simulink model "StateRequest"  (R2024a)
settings: Solver=FixedStepDiscrete  StartTime=0.0  StopTime=20  FixedStep=.005  RelTol=1e-3
values from neighbouring files (symbols this model uses):
  PrimaryState : value not decoded    [Dictionary.sldd]
libraries: simulink x4
settings Model: DataDictionary=Dictionary.sldd  Creator=aloehr  LastModifiedBy=aloehr
settings SolverCC: AlgebraicLoopSolver=TrustRegion  PositivePriorityOrder=on
settings OptimizationCC: DefaultParameterBehavior=Inlined  UseDivisionForNetSlopeComputation=on  GainParamInheritBuiltInType=on  UseFloatMulNetSlope=on  DefaultUnderspecifiedDataType=single  InlineInvariantSignals=on  PassReuseOutputArgsAs=Individual arguments  ZeroExternalMemoryAtStartup=off  ZeroInternalMemoryAtStartup=off  NoFixptDivByZeroProtection=on  EfficientFloat2IntCast=on  LifeSpan=1  MaxStackSize=64  OptimizeBlockOrder=speed  DifferentSizesBufferReuse=on  EfficientTunableParamExpr=on
settings DebuggingCC: ParameterTunabilityLossMsg=error  UnconnectedInputMsg=warning  UnconnectedOutputMsg=warning  UnconnectedLineMsg=warning  SFUnexpectedBacktrackingDiag=warning  SFNoUnconditionalDefaultTransitionDiag=warning
settings HardwareCC: ProdBitPerPointer=32  ProdBitPerSizeT=32  ProdBitPerPtrDiffT=32  ProdLargestAtomicInteger=Long  ProdLargestAtomicFloat=Double  ProdWordSize=32  ProdLongLongMode=on  ProdHWDeviceType=ARM Compatible->ARM Cortex-M  TargetBitPerPointer=64  TargetBitPerSizeT=64  TargetBitPerPtrDiffT=64  TargetLongLongMode=on  TargetIntDivRoundTo=Zero  TargetEndianess=LittleEndian  TargetWordSize=64  TargetHWDeviceType=MATLAB Host  ProdEqTarget=off
settings ModelReferenceCC: EnableRefExpFcnMdlSchedulingChecks=on
settings SFSimCC: MATLABDynamicMemAlloc=off
settings RTWCC: Description=Embedded Coder  SystemTargetFile=ert.tlc  GenCodeOnly=on  TemplateMakefile=ert_default_tmf  GenerateReport=on  Toolchain=GNU Tools for ARM Embedded Processors  BuildConfiguration=Debug  IncludeHyperlinkInReport=on  LaunchReport=on  DataTypeReplacement=CDataTypesFixedWidth  GenerateTraceInfo=on  GenerateTraceReport=on  GenerateTraceReportSl=on  GenerateTraceReportSf=on  GenerateTraceReportEml=on  GenerateCodeMetricsReport=on  GPUComputeCapability=3.5
settings CodeAppCC: ForceParamTrailComments=on  IgnoreCustomStorageClasses=off  OperatorAnnotations=on  SimulinkDataObjDesc=on  SFDataObjDesc=on  CustomSymbolStrGlobalVar=rt$N$M  CustomSymbolStrType=$N$M  CustomSymbolStrFcn=$N$M$F  CustomSymbolStrMacro=$N$M  InsertBlockDesc=on  EnableCustomComments=on  ReqsInCode=on
settings ERTTargetCC: TargetLangStandard=C99 (ISO)  CodeReplacementLibrary=GNU C99 extensions  GenerateSampleERTMain=on  IncludeMdlTerminateFcn=off  CombineSignalStateStructs=on  SupportAbsoluteTime=off  CodeInterfacePackaging=Reusable function  SupportComplex=off  SupportNonInlinedSFcns=on  InlinedParameterPlacement=NonHierarchical  ERTCustomFileTemplate=example_file_process.tlc  MaxIdInt64=INT64_MAX  MinIdInt64=INT64_MIN  MaxIdUint64=UINT64_MAX  MaxIdInt32=INT32_MAX  MinIdInt32=INT32_MIN  MaxIdUint32=UINT32_MAX  MaxIdInt16=INT16_MAX  MinIdInt16=INT16_MIN  MaxIdUint16=UINT16_MAX  MaxIdInt8=INT8_MAX  MinIdInt8=INT8_MIN  MaxIdUint8=UINT8_MAX

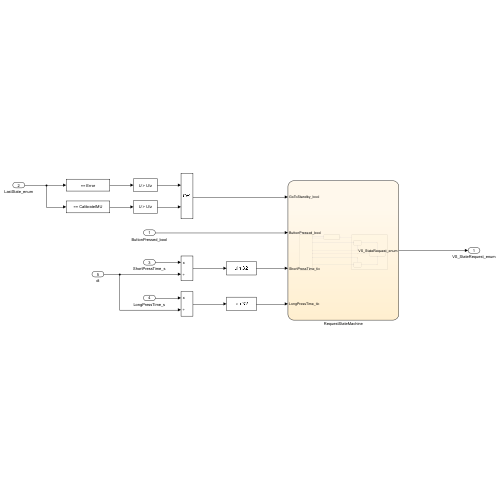
[thumbnail: Simulink's stored preview of the top-level diagram]
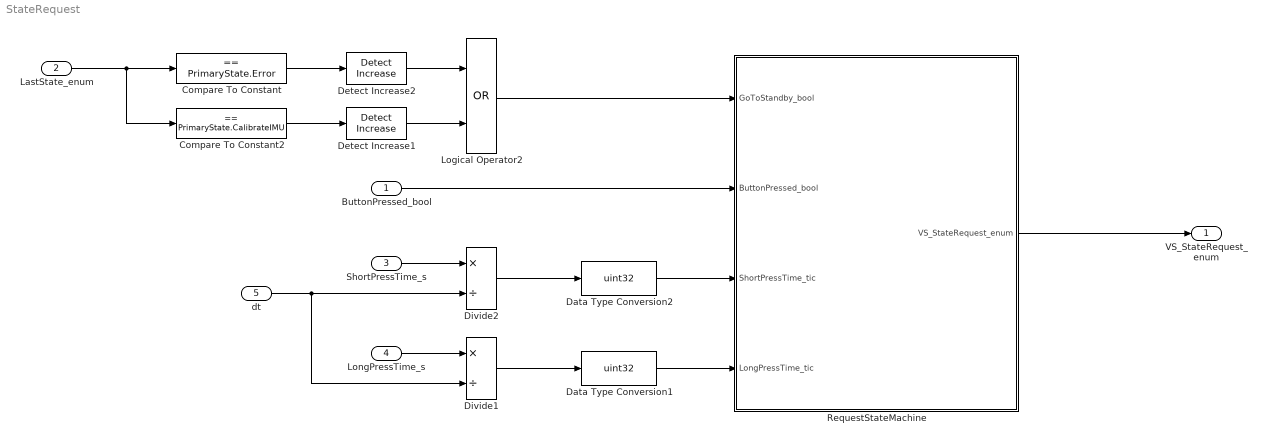
== system StateRequest ==
  ButtonPressed_bool : Inport  OutDataTypeStr=boolean
  LastState_enum : Inport  Port=2  OutDataTypeStr=Enum: PrimaryState
  ShortPressTime_s : Inport  Port=3  OutDataTypeStr=single
  LongPressTime_s : Inport  Port=4  OutDataTypeStr=single
  dt : Inport  Port=5  OutDataTypeStr=single
  Compare To Constant : simulink/Logic and Bit Operations/Compare To Constant  relop===  const=PrimaryState.Error  OutDataTypeStr=boolean
  Compare To Constant2 : simulink/Logic and Bit Operations/Compare To Constant  relop===  const=PrimaryState.CalibrateIMU  OutDataTypeStr=boolean
  Data Type Conversion1 : DataTypeConversion  OutDataTypeStr=uint32  SaturateOnIntegerOverflow=off  RndMeth=Floor
  Data Type Conversion2 : DataTypeConversion  OutDataTypeStr=uint32  SaturateOnIntegerOverflow=off  RndMeth=Floor
  Detect Increase1 : simulink/Logic and Bit Operations/Detect Increase  vinit=0.0  OutDataTypeStr=boolean
  Detect Increase2 : simulink/Logic and Bit Operations/Detect Increase  vinit=0.0  OutDataTypeStr=boolean
  Divide1 : Product  Inputs=*/
  Divide2 : Product  Inputs=*/
  Logical Operator2 : Logic  Operator=OR  AllPortsSameDT=off  OutDataTypeStr=boolean
  RequestStateMachine : Stateflow chart  TreatAsAtomicUnit=on
  VS_StateRequest_enum : Outport  OutDataTypeStr=Enum: StateReq
  wires:
  Compare To Constant2/1 -> Detect Increase1/1
  RequestStateMachine/1(VS_StateRequest_enum) -> VS_StateRequest_enum/1
  ButtonPressed_bool/1 -> RequestStateMachine/2(ButtonPressed_bool)
  LongPressTime_s/1 -> Divide1/1
  ShortPressTime_s/1 -> Divide2/1
  Detect Increase2/1 -> Logical Operator2/1
  Logical Operator2/1 -> RequestStateMachine/1(GoToStandby_bool)
  Divide1/1 -> Data Type Conversion1/1
  Data Type Conversion1/1 -> RequestStateMachine/4(LongPressTime_tic)
  Compare To Constant/1 -> Detect Increase2/1
  Data Type Conversion2/1 -> RequestStateMachine/3(ShortPressTime_tic)
  Divide2/1 -> Data Type Conversion2/1
  Detect Increase1/1 -> Logical Operator2/2
  LastState_enum/1 -> Compare To Constant/1, Compare To Constant2/1
  dt/1 -> Divide1/2, Divide2/2

== stateflow chart StateRequest/RequestStateMachine ==
  state NoCommand
  state GoToStandby
    VS_StateRequest_enum = StateReq.ReqStandby;
  state ButtonInput
    state Standby
    state CalibrateIMU
    state Balance
    Standby -> (junction 48) [order 1] : [after(LongPressTime_tic,tick)]
    (junction 48) -> CalibrateIMU
    Standby -> (junction 45) [order 2] : [after(ShortPressTime_tic,tick) && (~ButtonPressed_bool)]
    CalibrateIMU -> (junction 57) : [~ButtonPressed_bool]
    (junction 61) -> CalibrateIMU
    Balance -> (junction 52) [order 2] : [after(ShortPressTime_tic,tick) && (~ButtonPressed_bool)]
    Balance -> (junction 61) [order 1] : [after(LongPressTime_tic,tick)]
  (default) -> NoCommand : {VS_StateRequest_enum = StateReq.ReqStandby}
  NoCommand -> GoToStandby [order 1] : [GoToStandby_bool]
  ButtonInput -> GoToStandby : [GoToStandby_bool]
  GoToStandby -> NoCommand : [~GoToStandby_bool]
  NoCommand -> Standby [order 2] : [ButtonPressed_bool && (VS_StateRequest_enum == StateReq.ReqStandby)]
  (junction 45) -> NoCommand : {VS_StateRequest_enum = StateReq.ReqBalance}
  (junction 57) -> NoCommand : {VS_StateRequest_enum = StateReq.ReqCalibrateIMU}
  (junction 52) -> NoCommand : {VS_StateRequest_enum = StateReq.ReqStandby}
  NoCommand -> Balance [order 3] : [ButtonPressed_bool && (VS_StateRequest_enum == StateReq.ReqBalance)]
  data: GoToStandby_bool input boolean; ButtonPressed_bool input boolean; ShortPressTime_tic input uint32; VS_StateRequest_enum output Enum: StateReq =StateReq.ReqStandby; LongPressTime_tic input uint32
